simulink model "radar_system"  (R2021a)
settings: Solver=FixedStepDiscrete  StartTime=0.0  StopTime=1  RelTol=1e-3
PreLoadFcn:
  | load radar_system_var.mat;
  | radar_system_CarrierFreq = 2.1e9; % (Hz)
  | load radar_system_bjt.mat;
undefined symbols (not defined in the file): bitrevorder, dBc, findobj, Hz, M, radar_system_H, radar_system_L, radar_system_M, radar_system_N, radar_system_Nfft, radar_system_targetSpeed, radar_system_Ts, radar_system_wf
libraries: dspstat3 x10, dspmathops x6, dspmtrx3 x5, rfports1 x4, rfladderfilters1 x2, rfmixers1 x2, rfamplifiers1 x2, dspsrcs4 x2, dspxfrm3 x2, rfblackbox1 x1, commrflib2 x1, dspsigops x1
CloseFcn:
  | clear radar_system_*
settings Model: FPTRunName=Active  Creator=The MathWorks, Inc.  LastModifiedBy=kaka
settings SolverCC: AlgebraicLoopSolver=TrustRegion
settings DataIOCC: LimitDataPoints=on  SaveFormat=Array  SaveOutput=off  SignalLogging=off  SaveTime=off  ReturnWorkspaceOutputs=off
settings OptimizationCC: DefaultParameterBehavior=Inlined  ExpressionDepthLimit=2147483647  RollThreshold=2  InitFltsAndDblsToZero=on  LifeSpan=inf
settings DebuggingCC: AlgebraicLoopMsg=error  SaveWithParameterizedLinksMsg=none  UnderspecifiedInitializationDetection=Classic  MergeDetectMultiDrivingBlocksExec=none  SignalResolutionControl=TryResolveAllWithWarning  SolverPrmCheckMsg=warning  SingleTaskRateTransMsg=error  FcnCallInpInsideContextMsg=warning  StateNameClashWarn=warning  SFUnexpectedBacktrackingDiag=warning  SFNoUnconditionalDefaultTransitionDiag=warning  SFExecutionAtInitializationDiag=none  SFMachineParentedDataDiag=warning  ArithmeticOperatorsInVariantConditions=warning
settings HardwareCC: ProdBitPerPointer=32  ProdBitPerSizeT=32  ProdBitPerPtrDiffT=32  ProdLargestAtomicFloat=None  ProdIntDivRoundTo=Undefined  ProdEndianess=Unspecified  ProdWordSize=32  ProdHWDeviceType=32-bit Generic
settings ModelReferenceCC: PropagateSignalLabelsOutOfModel=off
settings SFSimCC: SimUseLocalCustomCode=off  SimParseCustomCode=off  CustomCodeUndefinedFunction=UseInterfaceOnly
settings RTWCC: RTWUseLocalCustomCode=off
settings CodeAppCC: StateflowObjectComments=on
settings GRTTargetCC: TargetFcnLib=ansi_tfl_tmw.mat  TargetLangStandard=C89/C90 (ANSI)  CombineOutputUpdateFcns=off  GRTInterface=on
settings ConfigComp: CovMetricSettings=dw  CovSaveCumulativeToWorkspaceVar=on  CovSaveSingleToWorkspaceVar=on  CovExternalEMLEnable=off  CovSFcnEnable=off

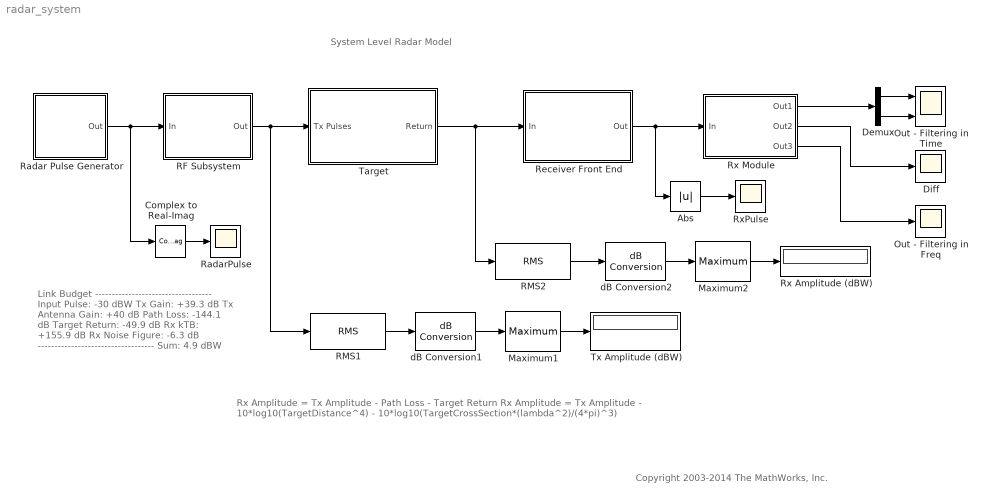
== system radar_system ==
  note: System Level Radar Model
  note: Rx Amplitude = Tx Amplitude - Path Loss - Target Return
      |
      | Rx Amplitude = Tx Amplitude - 10*log10(TargetDistance^4) - 10*log10(TargetCrossSection*(lambda^2)/(4*pi)^3)
  note: Link Budget
      | -----------------------------------
      | Input Pulse:            -30 dBW
      | Tx Gain:              +39.3 dB
      | Tx Antenna Gain:   +40 dB
      | Path Loss:         -144.1 dB
      | Target Return:     -49.9 dB
      | Rx kTB:             +155.9 dB
      | Rx Noise Figure:    -6.3 dB
      | -----------------------------------
      | Sum:                      4.9 dBW
  note: Copyright 2003-2014 The MathWorks, Inc.
  Abs : Abs
  Complex to Real-Imag : ComplexToRealImag  Output=Real
  Demux : Demux  Outputs=2
  Diff : Scope
  Maximum1 : dspstat3/Maximum  operation=maximum  fcn=Running  indexBase=One  operateOver=Each column  Dimension=1  InputProcessing=Columns as channels (frame based)  reset=None  roiEnable=off  roiType=Rectangles  roiPortion=Entire ROI  roiOutput=Individual statistics for each ROI  roiFlag=off  roundingMode=Floor  overflowMode=off  accumDataTypeStr=Inherit: Same as product output  accumLastDataTypeStr=Inherit: Same as product output
  Maximum2 : dspstat3/Maximum  operation=maximum  fcn=Running  indexBase=One  operateOver=Each column  Dimension=1  InputProcessing=Columns as channels (frame based)  reset=None  roiEnable=off  roiType=Rectangles  roiPortion=Entire ROI  roiOutput=Individual statistics for each ROI  roiFlag=off  roundingMode=Floor  overflowMode=off  accumDataTypeStr=Inherit: Same as product output  accumLastDataTypeStr=Inherit: Same as product output
  Out - Filtering in Freq : Scope
  Out - Filtering in Time : Scope  NumInputPorts=2
  RF Subsystem : Subsystem
  RMS1 : dspstat3/RMS  run=on  directionMode=Each column  dimension=1  InputProcessing=Columns as channels (frame based)  reset_popup=None
  RMS2 : dspstat3/RMS  run=on  directionMode=Each column  dimension=1  InputProcessing=Columns as channels (frame based)  reset_popup=None
  Radar Pulse Generator : Subsystem
  RadarPulse : Scope
  Receiver Front End : Subsystem
  Rx Amplitude (dBW) : Display
  Rx Module : Subsystem
  RxPulse : Scope
  Target : Subsystem  mask(Target){DistanceStart=4000, Speed=radar_system_targetSpeed, TargetCrossSection=1, Freq=radar_system_CarrierFreq}
      mask prompts: DistanceStart "Starting distance (m):"; Speed "Target speed (m/s):"; TargetCrossSection "Target cross section (m^2):"; Freq "Carrier frequency (Hz):"
      mask init:
      | Wavelength=3e8/Freq;      % Speed/Frequency;
      | Doppler=Speed/Wavelength; % Doppler shift Vehicle speed/Wavelength
  Tx Amplitude (dBW) : Display
  dB Conversion1 : dspmathops/dB Conversion  dBtype=dB  intype=Amplitude  R=1  fuzz=on
  dB Conversion2 : dspmathops/dB Conversion  dBtype=dB  intype=Amplitude  R=1  fuzz=on
  wires:
  Radar Pulse Generator/1(Out) -> RF Subsystem/1(In), Complex to Real-Imag/1
  Target/1(Return) -> Receiver Front End/1(In), RMS2/1
  RF Subsystem/1(Out) -> RMS1/1, Target/1(Tx Pulses)
  dB Conversion1/1 -> Maximum1/1
  RMS2/1 -> dB Conversion2/1
  dB Conversion2/1 -> Maximum2/1
  Receiver Front End/1(Out) -> Rx Module/1(In), Abs/1
  Rx Module/2(Out2) -> Diff/1
  Rx Module/3(Out3) -> Out - Filtering in Freq/1
  Rx Module/1(Out1) -> Demux/1
  Demux/1 -> Out - Filtering in Time/1
  Demux/2 -> Out - Filtering in Time/2
  Complex to Real-Imag/1 -> RadarPulse/1
  Abs/1 -> RxPulse/1
  RMS1/1 -> dB Conversion1/1
  Maximum1/1 -> Tx Amplitude (dBW)/1
  Maximum2/1 -> Rx Amplitude (dBW)/1

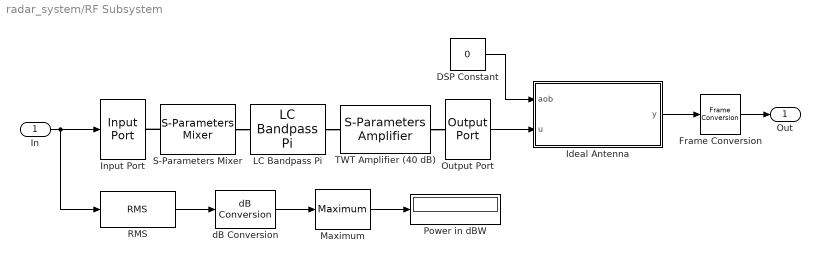
== system radar_system/RF Subsystem ==
  In : Inport
  DSP Constant : Constant  Value=0  VectorParams1D=off  SampleTime=radar_system_Ts
  Frame Conversion : FrameConversion  OutFrame=Sample-based
  Ideal Antenna : Subsystem  InitFcn=close(findobj('Tag','PointingLossULANull'))  mask(Ideal Antenna){G=40}
      mask prompts: G "Antenna gain (dB):"
      settings: CloseFcn=close(findobj('Tag','PointingLossULANull'))
  Input Port : rfports1/Input Port  Description=source block  TreatSimulinkInputSignalAs=Incident power wave  MaxLength=128  FracBW=0  ModelDelay=0  Fc=radar_system_CarrierFreq  Ts=radar_system_Ts/8  Zs=50  RFhasDSP=Columns as channels (frame based)  NoiseFlag=off  seed=67987  GoToTag=BAEGAKNGGHPPZNUZGFDAKSO
      settings: SourceProductBaseCode=RB
  LC Bandpass Pi : rfladderfilters1/LC Bandpass Pi  LConnTagsString=__newl0  RConnTagsString=__newr0  L="[1.4446e-9  4.3949e-8  1.4446e-9]*.32"  C="[3.5785e-11  1.1762e-12  3.5785e-11]*.32"  PlotFreq=User-specified  SourceFreq=User-specified  Freq=[1000e6:4e6:3000e6]  AllPlotType=X-Y plane  AppliedNetworkData=S21  AppliedComplexFormat=Magnitude (decibels)  AppliedNetworkData2=""  AppliedXParameter=Freq  AppliedXFormat=Hz  YOption=Linear  XOption=Linear  PlotZ0=50  DisplayData=off  PlotFreqNoSim=User-specified  NetworkData=S21  SmithData=S11  PolarData=S11  ComplexFormat=Magnitude (decibels)  DBFormat=Magnitude (decibels)  NoneFormat=None
      settings: SourceProductBaseCode=RB
  Maximum : dspstat3/Maximum  operation=maximum  fcn=Running  indexBase=One  operateOver=Each column  Dimension=1  reset=None  roiEnable=off  roiType=Rectangles  roiPortion=Entire ROI  roiOutput=Individual statistics for each ROI  roiFlag=off  roundingMode=Floor  overflowMode=off  accumDataTypeStr=Inherit: Same as product output  accumLastDataTypeStr=Inherit: Same as product output
  Output Port : rfports1/Output Port  Zl=50  Flag=1  num_Models=0  GoToTag=BAEGAKNGGHPPZNUZGFDAKSO  PlotFreq=User-specified  SourceFreq=Derived from Input Port parameters  Freq=1e9:1e8:3e9  AllPlotType=X-Y plane  AppliedNetworkData=S21  AppliedComplexFormat=Magnitude (decibels)  AppliedNetworkData2=""  AppliedComplexFormat2=""  AppliedXParameter=Freq  AppliedXFormat=Hz  YOption=Linear  XOption=Linear  PlotZ0=50  DisplayData=off  NoBudgetPlot=Composite data  NetworkData=S11  SmithData=S11  PolarData=S11  ComplexFormat=Magnitude (decibels)  DBFormat=Magnitude (decibels)  DBMFormat=dBm  NoneFormat=None
      settings: SourceProductBaseCode=RB
  Power in dBW : Display
  RMS : dspstat3/RMS  run=off  directionMode=Each column  dimension=1  InputProcessing=Columns as channels (frame based)  reset_popup=None
  S-Parameters Mixer : rfmixers1/S-Parameters Mixer  LConnTagsString=__newl0  RConnTagsString=__newr0  NetParamData=[0 0;1 0]  NetParamFreq=radar_system_CarrierFreq  Z0=50  InterpMethod=Linear  MixerType=Upconverter  FLO=0  IP3Type=OIP3  IIP3=inf  OIP3=inf  P1dB=inf  PSat=inf  GCSat=0  NonlinearDataFreq=2.0e9  NoiseDefinedBy=Noise figure  NF=0  FMIN=0  GammaOpt=1  RN=1  NFactor=1  NTemp=0  NoiseDataFreq=2.0e9  FreqOffset=[0.1 1 10 100]*1e3  PhaseNoiseLevel=[-70 -120 -140 -150]  PlotFreq=Same as the Frequency parameter  SourceFreq=Same as the s-parameters frequency  Freq=[1e9:1e8:2.9e9]  SourcePin=Extracted from data source  Pin=0  AllPlotType=X-Y plane  AppliedNetworkData=S11  AppliedComplexFormat=Magnitude (decibels)  AppliedNetworkData2=""  AppliedComplexFormat2=""  AppliedXParameter=Freq  AppliedXFormat=Auto  YOption=Linear  XOption=Linear  PlotZ0=50  PlotFreqNoSim=0  DisplayData=0  NetworkData=0  SmithData=0  PolarData=0  ComplexFormat=0  DBFormat=0  NoneFormat=0  DBcFormat=0
      settings: SourceProductBaseCode=RB
  TWT Amplifier (40 dB) : rfamplifiers1/S-Parameters Amplifier  LConnTagsString=__newl0  RConnTagsString=__newr0  NetParamData=[0,0;sqrt(10000),0]  NetParamFreq=radar_system_CarrierFreq  Z0=50  InterpMethod=Linear  IP3Type=OIP3  IIP3=50  OIP3=50  P1dB=inf  PSat=inf  GCSat=0  NonlinearDataFreq=2.0e9  NoiseDefinedBy=Noise figure  NF=8  FMIN=0  GammaOpt=1  RN=1  NFactor=1  NTemp=0  NoiseDataFreq=2.0e9  PlotFreq=Derived from Input Port parameters  SourceFreq=Same as the s-parameters frequency  Freq=[1.9e9:1.0e8:2.2e9]  SourcePin=Extracted from data source  Pin=0  AllPlotType=X-Y plane  AppliedNetworkData=S11  AppliedComplexFormat=Magnitude (decibels)  AppliedNetworkData2=""  AppliedComplexFormat2=""  AppliedXParameter=Freq  AppliedXFormat=Auto  YOption=Linear  XOption=Linear  PlotZ0=50  PlotFreqNoSim=0  DisplayData=0  NetworkData=0  SmithData=0  PolarData=0  ComplexFormat=0  DBFormat=0  NoneFormat=0
      settings: SourceProductBaseCode=RB
  dB Conversion : dspmathops/dB Conversion  dBtype=dB  intype=Amplitude  R=1  fuzz=on
  Out : Outport  VectorParamsAs1DForOutWhenUnconnected=off
  wires:
  Output Port/1 -> Ideal Antenna/2(u)
  In/1 -> RMS/1, Input Port/1
  Frame Conversion/1 -> Out/1
  Maximum/1 -> Power in dBW/1
  RMS/1 -> dB Conversion/1
  dB Conversion/1 -> Maximum/1
  Ideal Antenna/1(y) -> Frame Conversion/1
  DSP Constant/1 -> Ideal Antenna/1(aob)
  connections:
  LC Bandpass Pi/RConn1 -- TWT Amplifier (40 dB)/LConn1
  TWT Amplifier (40 dB)/RConn1 -- Output Port/LConn1
  S-Parameters Mixer/LConn1 -- Input Port/RConn1
  S-Parameters Mixer/RConn1 -- LC Bandpass Pi/LConn1

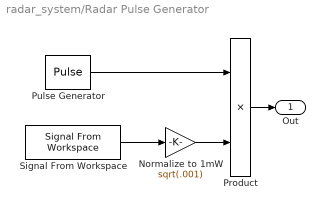
== system radar_system/Radar Pulse Generator ==
  Normalize to 1mW : Gain  Gain=sqrt(.001)
  Product : Product  RndMeth=Zero
  Pulse Generator : DiscretePulseGenerator  Period=50*length(radar_system_wf)  PulseWidth=length(radar_system_wf)  SampleTime=radar_system_Ts/8
  Signal From Workspace : dspsrcs4/Signal From Workspace  X=radar_system_wf  Ts=radar_system_Ts/8  nsamps=1  OutputAfterFinalValue=Cyclic repetition  ignoreOrWarnInputAndFrameLengths=off  OutputFrames=on
  Out : Outport  VectorParamsAs1DForOutWhenUnconnected=off
  wires:
  Normalize to 1mW/1 -> Product/2
  Signal From Workspace/1 -> Normalize to 1mW/1
  Pulse Generator/1 -> Product/1
  Product/1 -> Out/1

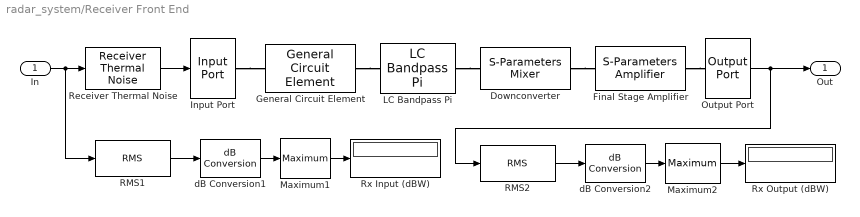
== system radar_system/Receiver Front End ==
  In : Inport
  Downconverter : rfmixers1/S-Parameters Mixer  LConnTagsString=__newl0  RConnTagsString=__newr0  NetParamData=[0,0;.5,0]  NetParamFreq=radar_system_CarrierFreq  Z0=50  InterpMethod=Linear  MixerType=Downconverter  FLO=radar_system_CarrierFreq - 70e6  IP3Type=OIP3  IIP3=inf  OIP3=100  P1dB=inf  PSat=inf  GCSat=0  NonlinearDataFreq=2.0e9  NoiseDefinedBy=Noise figure  NF=5  FMIN=0  GammaOpt=1  RN=1  NFactor=1  NTemp=0  NoiseDataFreq=2.0e9  FreqOffset=[0.1 1 10 100]*1e3  PhaseNoiseLevel=[-70 -120 -140 -150]  PlotFreq=Derived from Input Port parameters  SourceFreq=Same as the s-parameters frequency  Freq=[1.9e9:1.0e8:2.2e9]  SourcePin=Extracted from data source  Pin=0  AllPlotType=X-Y plane  AppliedNetworkData=S11  AppliedComplexFormat=Magnitude (decibels)  AppliedNetworkData2=""  AppliedComplexFormat2=""  AppliedXParameter=Freq  AppliedXFormat=Auto  YOption=Linear  XOption=Linear  PlotZ0=50  PlotFreqNoSim=Same as the Frequency parameter  DisplayData=off  NetworkData=S21  SmithData=S11  PolarData=S12  ComplexFormat=Magnitude (decibels)  DBFormat=Magnitude (decibels)  NoneFormat=None  DBcFormat=dBc/Hz
      settings: SourceProductBaseCode=RB
  Final Stage Amplifier : rfamplifiers1/S-Parameters Amplifier  LConnTagsString=__newl0  RConnTagsString=__newr0  NetParamData=[0,0;sqrt(1000),0]  NetParamFreq=70e6  Z0=50  InterpMethod=Linear  IP3Type=OIP3  IIP3=-10  OIP3=100  P1dB=inf  PSat=inf  GCSat=0  NonlinearDataFreq=2.0e9  NoiseDefinedBy=Noise figure  NF=8  FMIN=0  GammaOpt=1  RN=1  NFactor=1  NTemp=0  NoiseDataFreq=2.0e9  PlotFreq=Derived from Input Port parameters  SourceFreq=Same as the s-parameters frequency  Freq=[1.9e9:1.0e8:2.2e9]  SourcePin=Extracted from data source  Pin=0  AllPlotType=ZY Smith chart  AppliedNetworkData=S11  AppliedComplexFormat=Magnitude (decibels)  AppliedNetworkData2=""  AppliedXParameter=Freq  AppliedXFormat=Hz  YOption=Linear  XOption=Linear  PlotZ0=50  PlotFreqNoSim=Same as the Frequency parameter  DisplayData=off  NetworkData=S21  SmithData=S11  PolarData=S12  ComplexFormat=Magnitude (decibels)  DBFormat=Magnitude (decibels)  NoneFormat=None
      settings: SourceProductBaseCode=RB
  General Circuit Element : rfblackbox1/General  Circuit Element  LConnTagsString=__newl0  RConnTagsString=__newr0  Ckt=radar_system_bjt  PlotFreq=User-specified  SourceFreq=User-specified  Freq=[1.9e9:1.0e6:2.2e9]  AllPlotType=X-Y plane  AppliedNetworkData=S22  AppliedComplexFormat=Magnitude (decibels)  AppliedNetworkData2=""  AppliedComplexFormat2=""  AppliedXParameter=Freq  AppliedXFormat=Hz  YOption=Linear  XOption=Linear  PlotZ0=50  PlotFreqNoSim=User-specified  DisplayData=off  NetworkData=S21  SmithData=S11  PolarData=S11  ComplexFormat=Magnitude (decibels)  DBFormat=Magnitude (decibels)  NoneFormat=None
      settings: SourceProductBaseCode=RB
  Input Port : rfports1/Input Port  Description=source block  TreatSimulinkInputSignalAs=Incident power wave  MaxLength=128  FracBW=0  ModelDelay=0  Fc=radar_system_CarrierFreq  Ts=radar_system_Ts/8  Zs=50  RFhasDSP=Columns as channels (frame based)  NoiseFlag=on  seed=67987  GoToTag=AABCIBALDJCBLQNCZTQCBHN
      settings: SourceProductBaseCode=RB
  LC Bandpass Pi : rfladderfilters1/LC Bandpass Pi  LConnTagsString=__newl0  RConnTagsString=__newr0  L="[1.4446e-9  4.3949e-8  1.4446e-9]*.32"  C="[3.5785e-11  1.1762e-12  3.5785e-11]*.32"  PlotFreq=User-specified  SourceFreq=User-specified  Freq=[1000e6:4e6:3000e6]  AllPlotType=X-Y plane  AppliedNetworkData=S21  AppliedComplexFormat=Magnitude (decibels)  AppliedNetworkData2=""  AppliedXParameter=Freq  AppliedXFormat=Hz  YOption=Linear  XOption=Linear  PlotZ0=50  DisplayData=off  PlotFreqNoSim=User-specified  NetworkData=S21  SmithData=S11  PolarData=S11  ComplexFormat=Magnitude (decibels)  DBFormat=Magnitude (decibels)  NoneFormat=None
      settings: SourceProductBaseCode=RB
  Maximum1 : dspstat3/Maximum  operation=maximum  fcn=Running  indexBase=One  operateOver=Each column  Dimension=1  reset=None  roiEnable=off  roiType=Rectangles  roiPortion=Entire ROI  roiOutput=Individual statistics for each ROI  roiFlag=off  roundingMode=Floor  overflowMode=off  accumDataTypeStr=Inherit: Same as product output  accumLastDataTypeStr=Inherit: Same as product output
  Maximum2 : dspstat3/Maximum  operation=maximum  fcn=Running  indexBase=One  operateOver=Each column  Dimension=1  reset=None  roiEnable=off  roiType=Rectangles  roiPortion=Entire ROI  roiOutput=Individual statistics for each ROI  roiFlag=off  roundingMode=Floor  overflowMode=off  accumDataTypeStr=Inherit: Same as product output  accumLastDataTypeStr=Inherit: Same as product output
  Output Port : rfports1/Output Port  Zl=50  Flag=0  num_Models=0  GoToTag=AABCIBALDJCBLQNCZTQCBHN  PlotFreq=User-specified  SourceFreq=Derived from Input Port parameters  Freq=1e9:1e8:3e9  AllPlotType=X-Y plane  AppliedNetworkData=S21  AppliedComplexFormat=Magnitude (decibels)  AppliedNetworkData2=NF  AppliedComplexFormat2=Magnitude (decibels)  AppliedXParameter=Freq  AppliedXFormat=Hz  YOption=Linear  XOption=Linear  PlotZ0=50  DisplayData=off  NoBudgetPlot=Composite data  NetworkData=S11  SmithData=S11  PolarData=S11  ComplexFormat=Magnitude (decibels)  DBFormat=Magnitude (decibels)  DBMFormat=dBm  NoneFormat=None
      settings: SourceProductBaseCode=RB
  RMS1 : dspstat3/RMS  run=on  directionMode=Each column  dimension=1  reset_popup=None
  RMS2 : dspstat3/RMS  run=on  directionMode=Each column  dimension=1  reset_popup=None
  Receiver Thermal Noise : commrflib2/Receiver Thermal Noise  method=Noise temperature  ntemp=290  nfigure=3.01  nfactor=2  add290KAntennaNoise=off  seed=67987
      settings: SourceProductBaseCode=CM
  Rx Input (dBW) : Display
  Rx Output (dBW) : Display
  dB Conversion1 : dspmathops/dB Conversion  dBtype=dB  intype=Amplitude  R=1  fuzz=on
  dB Conversion2 : dspmathops/dB Conversion  dBtype=dB  intype=Amplitude  R=1  fuzz=on
  Out : Outport  VectorParamsAs1DForOutWhenUnconnected=off
  wires:
  In/1 -> RMS1/1, Receiver Thermal Noise/1
  Output Port/1 -> Out/1, RMS2/1
  dB Conversion1/1 -> Maximum1/1
  RMS1/1 -> dB Conversion1/1
  dB Conversion2/1 -> Maximum2/1
  RMS2/1 -> dB Conversion2/1
  Maximum1/1 -> Rx Input (dBW)/1
  Maximum2/1 -> Rx Output (dBW)/1
  Receiver Thermal Noise/1 -> Input Port/1
  connections:
  Final Stage Amplifier/RConn1 -- Output Port/LConn1
  Input Port/RConn1 -- General Circuit Element/LConn1
  Downconverter/RConn1 -- Final Stage Amplifier/LConn1
  General Circuit Element/RConn1 -- LC Bandpass Pi/LConn1
  LC Bandpass Pi/RConn1 -- Downconverter/LConn1

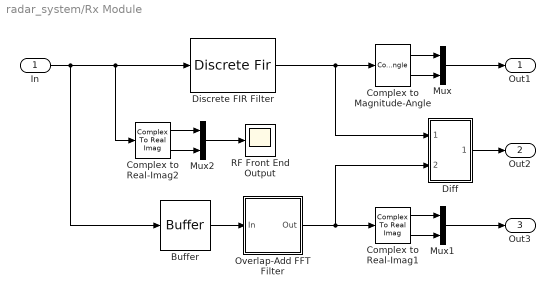
== system radar_system/Rx Module ==
  In : Inport
  Buffer : Buffer  N=radar_system_Nfft
  Complex to Magnitude-Angle : ComplexToMagnitudeAngle
  Complex to Real-Imag1 : ComplexToRealImag
  Complex to Real-Imag2 : ComplexToRealImag
  Diff : Subsystem
  Discrete FIR Filter : DiscreteFir  Coefficients=fliplr(radar_system_wf)  InitialStates=eps  AccumDataTypeStr=Inherit: Same as product output
  Mux : Mux  Inputs=2
  Mux1 : Mux  Inputs=2
  Mux2 : Mux  Inputs=2
  Overlap-Add FFT Filter : Subsystem
  RF Front End Output : Scope
  Out1 : Outport  VectorParamsAs1DForOutWhenUnconnected=off
  Out2 : Outport  Port=2  VectorParamsAs1DForOutWhenUnconnected=off
  Out3 : Outport  Port=3  VectorParamsAs1DForOutWhenUnconnected=off
  wires:
  Complex to Magnitude-Angle/1 -> Mux/1
  Complex to Magnitude-Angle/2 -> Mux/2
  Discrete FIR Filter/1 -> Diff/1(In1), Complex to Magnitude-Angle/1
  Mux/1 -> Out1/1
  Complex to Real-Imag1/1 -> Mux1/1
  Complex to Real-Imag1/2 -> Mux1/2
  Overlap-Add FFT Filter/1(Out) -> Complex to Real-Imag1/1, Diff/2(In2)
  Mux1/1 -> Out3/1
  Buffer/1 -> Overlap-Add FFT Filter/1(In)
  In/1 -> Discrete FIR Filter/1, Complex to Real-Imag2/1, Buffer/1
  Complex to Real-Imag2/1 -> Mux2/1
  Complex to Real-Imag2/2 -> Mux2/2
  Diff/1(Out1) -> Out2/1
  Mux2/1 -> RF Front End Output/1

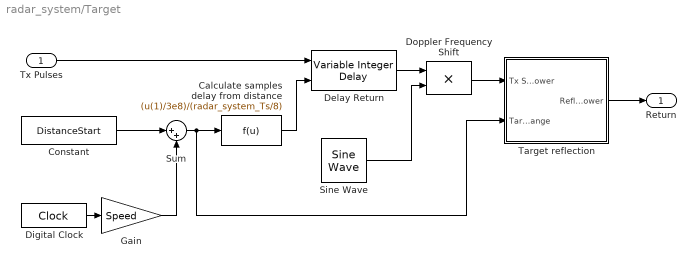
== system radar_system/Target ==
  Tx Pulses : Inport
  Calculate samples delay from distance : Fcn  Expr=(u(1)/3e8)/(radar_system_Ts/8)
  Constant : Constant  Value=DistanceStart
  Delay Return : dspobslib/Variable Integer Delay  dmax=100  ic=0  noDFT=off
      settings: SourceProductBaseCode=DS
  Digital Clock : DigitalClock  SampleTime=radar_system_Ts/8
  Doppler Frequency Shift : Product  InputSameDT=on  SaturateOnIntegerOverflow=on  OutDataTypeStr=Inherit: Same as first input
  Gain : Gain  Gain=Speed  SaturateOnIntegerOverflow=on  OutDataTypeStr=Inherit: Same as input  ParamDataTypeStr=Inherit: Same as input
  Sine Wave : dspsrcs4/Sine Wave  Amplitude=1  Frequency=(Doppler+eps)  Phase=0  SampleMode=Discrete  OutComplex=Complex  CompMethod=Trigonometric fcn  TableSize=Speed  SampleTime=radar_system_Ts/8  SamplesPerFrame=1  ResetState=Restart at time zero  OutputFrames=on  dataType=double  wordLen=16  udDataType=sfix(16)  fracBitsMode=Best precision  numFracBits=14  OutDataTypeStr=double  LastOutDataTypeStr=double
  Sum : Sum  Inputs=|++  InputSameDT=on  SaturateOnIntegerOverflow=on  OutDataTypeStr=Inherit: Same as first input
  Target reflection : Subsystem  mask{sigma=TargetCrossSection, lambda=Wavelength}
      mask prompts: sigma "Target RCS (m^2):"; lambda "Wavelength of Radar (m):"
  Return : Outport  VectorParamsAs1DForOutWhenUnconnected=off
  wires:
  Target reflection/1(Reflected Power) -> Return/1
  Doppler Frequency Shift/1 -> Target reflection/1(Tx Signal Power)
  Sum/1 -> Calculate samples delay from distance/1, Target reflection/2(Target Range)
  Constant/1 -> Sum/1
  Gain/1 -> Sum/2
  Digital Clock/1 -> Gain/1
  Calculate samples delay from distance/1 -> Delay Return/2
  Delay Return/1 -> Doppler Frequency Shift/1
  Tx Pulses/1 -> Delay Return/1
  Sine Wave/1 -> Doppler Frequency Shift/2

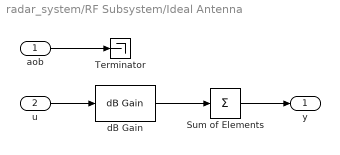
== system radar_system/RF Subsystem/Ideal Antenna ==
  aob : Inport
  u : Inport  Port=2
  Sum of Elements : Sum  Inputs=+
  Terminator : Terminator
  dB Gain : dspmathops/dB Gain  dB=G  intype=Amplitude
      settings: SourceProductBaseCode=DS
  y : Outport  VectorParamsAs1DForOutWhenUnconnected=off
  wires:
  Sum of Elements/1 -> y/1
  dB Gain/1 -> Sum of Elements/1
  aob/1 -> Terminator/1
  u/1 -> dB Gain/1

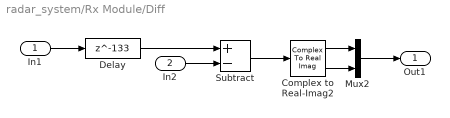
== system radar_system/Rx Module/Diff ==
  In1 : Inport
  In2 : Inport  Port=2
  Complex to Real-Imag2 : ComplexToRealImag
  Delay : Delay  DelayLength=133  InitialCondition=0
  Mux2 : Mux  Inputs=2
  Subtract : Sum  Inputs=+-
  Out1 : Outport  VectorParamsAs1DForOutWhenUnconnected=off
  wires:
  Complex to Real-Imag2/1 -> Mux2/1
  Complex to Real-Imag2/2 -> Mux2/2
  Mux2/1 -> Out1/1
  Subtract/1 -> Complex to Real-Imag2/1
  Delay/1 -> Subtract/1
  In1/1 -> Delay/1
  In2/1 -> Subtract/2

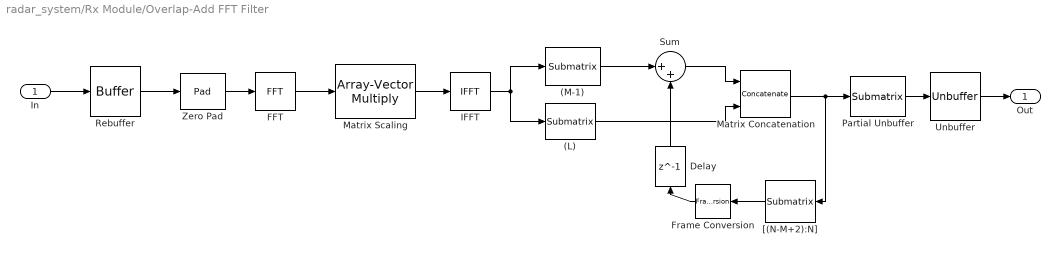
== system radar_system/Rx Module/Overlap-Add FFT Filter ==
  In : Inport
  (L) : dspmtrx3/Submatrix  RowSpan=Range of rows  RowStartMode=Offset from last  RowStartIndex=radar_system_L-1  RowEndMode=Last  RowEndIndex=1  ColSpan=All columns  ColStartMode=First  ColStartIndex=1  ColEndMode=Last  ColEndIndex=1
  (M-1) : dspmtrx3/Submatrix  RowSpan=Range of rows  RowStartMode=First  RowStartIndex=M-1  RowEndMode=Index  RowEndIndex=radar_system_M-1  ColSpan=All columns  ColStartMode=First  ColStartIndex=1  ColEndMode=Last  ColEndIndex=1
  Delay : Delay  DelayLength=1  InitialCondition=0  UseCircularBuffer=on
  FFT : dspxfrm3/FFT  FFTImplementation=Auto  CompMethod=Table lookup  TableOpt=NEW  TableOptActive=Speed  BitRevOrder=on  Normalize=on  InheritFFTLength=on  FFTLength=64  WrapInput=on  roundingMode=Floor  overflowMode=off  firstCoeffDataTypeStr=Inherit: Same word length as input  firstCoeffLastDataTypeStr=Inherit: Same word length as input  outputMin=[]  outputMax=[]
  Frame Conversion : FrameConversion  OutFrame=Sample-based
  IFFT : dspxfrm3/IFFT  FFTImplementation=Auto  CompMethod=Table lookup  TableOpt=NEW  TableOptActive=Speed  BitRevOrder=on  cs_in=off  Normalize=off  InheritFFTLength=on  FFTLength=64  WrapInput=on  mode=Complex  outSamplingMode=Frame based  roundingMode=Floor  overflowMode=off  firstCoeffDataTypeStr=Inherit: Same word length as input  firstCoeffLastDataTypeStr=Inherit: Same word length as input  outputMin=[]  outputMax=[]
  Matrix Concatenation : Concatenate  Mode=Multidimensional array
  Matrix Scaling : dspmtrx3/Array-Vector Multiply  mode=Mute  saveAsFlag=0  Dimension=1  V_Source=Dialog parameter  V_VectFromMask=bitrevorder(radar_system_H(:))  roundingMode=Floor  overflowMode=off  firstCoeffMode=Binary point scaling  firstCoeffSignedness=Auto  firstCoeffWordLength=16  firstCoeffFracLength=11  firstCoeffDataTypeStr=fixdt(1,16,11)  firstCoeffMin=[]  firstCoeffMax=[]  firstCoeffLastDataTypeStr=fixdt(1,16,11)  prodOutputMode=Binary point scaling  prodOutputSignedness=Auto  prodOutputWordLength=32  prodOutputFracLength=23  prodOutputDataTypeStr=fixdt([],32,23)  prodOutputLastDataTypeStr=fixdt([],32,23)  accumMode=Binary point scaling  accumSignedness=Auto  accumWordLength=32  accumFracLength=23  accumDataTypeStr=fixdt([],32,23)  accumLastDataTypeStr=fixdt([],32,23)  outputMode=Binary point scaling  outputSignedness=Auto  outputWordLength=16  outputFracLength=7  outputDataTypeStr=fixdt([],16,7)  outputMin=[]  outputMax=[]  outputLastDataTypeStr=fixdt([],16,7)
      settings: SourceProductBaseCode=DS  allowOverrides=off
  Partial Unbuffer : dspmtrx3/Submatrix  RowSpan=Range of rows  RowStartMode=First  RowStartIndex=M  RowEndMode=Index  RowEndIndex=radar_system_L  ColSpan=All columns  ColStartMode=First  ColStartIndex=1  ColEndMode=Last  ColEndIndex=1
  Rebuffer : Buffer  N=radar_system_L
  Sum : Sum  Inputs=|++
  Unbuffer : Unbuffer
  Zero Pad : dspsigops/Pad  padAlong=Columns  dimsToPad=1  valSrc=Specify via dialog  padVal=0  spec=Output size  padNumOutRowsSpecMethod=User-specified  numOutRows=radar_system_N  padNumOutColsSpecMethod=User-specified  numOutCols=1  isVarDimsMode=off  padBeginning=0  padEnd=0  outSizeMode=User-specified  outSize=1  padSigAt=End  trunc_flag=None  roundingMode=Floor  overflowMode=off  truncOrWrapMode=Truncate  wrap_flag=None
      settings: SourceProductBaseCode=DS
  "[(N-M+2):N]" : dspmtrx3/Submatrix  RowSpan=Range of rows  RowStartMode=Index  RowStartIndex=(radar_system_N-radar_system_M+2)  RowEndMode=Last  RowEndIndex=N  ColSpan=All columns  ColStartMode=First  ColStartIndex=1  ColEndMode=Last  ColEndIndex=1
  Out : Outport  VectorParamsAs1DForOutWhenUnconnected=off
  wires:
  In/1 -> Rebuffer/1
  FFT/1 -> Matrix Scaling/1
  Rebuffer/1 -> Zero Pad/1
  Zero Pad/1 -> FFT/1
  IFFT/1 -> (M-1)/1, (L)/1
  Matrix Scaling/1 -> IFFT/1
  Unbuffer/1 -> Out/1
  Matrix Concatenation/1 -> "[(N-M+2):N]"/1, Partial Unbuffer/1
  "[(N-M+2):N]"/1 -> Frame Conversion/1
  (L)/1 -> Matrix Concatenation/2
  Delay/1 -> Sum/2
  (M-1)/1 -> Sum/1
  Sum/1 -> Matrix Concatenation/1
  Partial Unbuffer/1 -> Unbuffer/1
  Frame Conversion/1 -> Delay/1

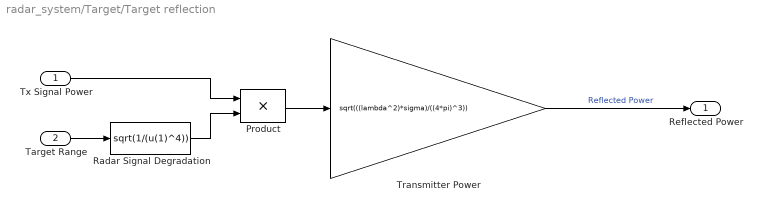
== system radar_system/Target/Target reflection ==
  Tx Signal Power : Inport
  Target Range : Inport  Port=2
  Product : Product  InputSameDT=on  SaturateOnIntegerOverflow=on  OutDataTypeStr=Inherit: Same as first input
  Radar Signal Degradation : Fcn  Expr=sqrt(1/(u(1)^4))
  Transmitter Power : Gain  Gain=sqrt(((lambda^2)*sigma)/((4*pi)^3))  SaturateOnIntegerOverflow=on  OutDataTypeStr=Inherit: Same as input  ParamDataTypeStr=Inherit: Same as input
  Reflected Power : Outport  VectorParamsAs1DForOutWhenUnconnected=off
  wires:
  Transmitter Power/1 -> Reflected Power/1  "Reflected Power"
  Product/1 -> Transmitter Power/1
  Tx Signal Power/1 -> Product/1
  Target Range/1 -> Radar Signal Degradation/1
  Radar Signal Degradation/1 -> Product/2
